simulink model "EV3_pos_control"  (Simulink 9.2)
settings: Solver=FixedStepDiscrete  StartTime=0.0  StopTime=Inf  RelTol=1e-3  EnableMultiTasking=on
InitFcn:
  | nxt_rst
values from neighbouring files (symbols this model uses):
  R = double(vpa(coeffs(collect(expand(eval(Ax*R0))),z_),Acc))    [nxt_rst.m]
  S = double(vpa(coeffs(collect(expand(eval((1-z_)^p*Bx*S2))),z_),Acc))    [nxt_rst.m]
  T = double(vpa(coeffs(collect(expand(eval(Ax*T0))),z_),Acc))    [nxt_rst.m]
  Te = 0.01    [init_ident.m]    (also in nxt_rst.m)
undefined symbols (not defined in the file or in its folder): adjustCoefficients
libraries: rpi_blkst x1
settings Model: Creator=jacques  LastModifiedBy=jacques  SimulationMode=external
settings OptimizationCC: ExpressionDepthLimit=2147483647  LifeSpan=1
settings DebuggingCC: SolverPrmCheckMsg=warning
settings HardwareCC: ProdLargestAtomicInteger=Long  ProdLargestAtomicFloat=Double  ProdIntDivRoundTo=Zero  ProdEndianess=LittleEndian  ProdHWDeviceType=ARM Compatible->ARM Cortex
settings SFSimCC: MATLABDynamicMemAlloc=off
settings RTWCC: SystemTargetFile=ert_rpi.tlc  TemplateMakefile=ert_rpi.tmf  PostCodeGenCommand=postGenFunc(buildInfo)  Description=RTW Embedded Coder RPI target
settings CodeAppCC: IgnoreCustomStorageClasses=off  CustomSymbolStrType=$N$R$M  InternalIdentifier=Classic
settings STFCustomTargetCC: ModelReferenceCompliant=off  CombineOutputUpdateFcns=on  ERTCustomFileBanners=on  SupportNonInlinedSFcns=off  RemoveResetFunc=on  MATLABClassNameForMDSCustomization=Simulink.SoftwareTarget.ERTCustomization  GRTInterface=off  SystemTargetFile=ert_rpi.tlc
settings ERTTargetCC: MultiwordLength=2048  ModelReferenceCompliant=off  ParMdlRefBuildCompliant=off  CompOptLevelCompliant=off  ConcurrentExecutionCompliant=off  SupportContinuousTime=on  ModelStepFunctionPrototypeControlCompliant=off  CPPClassGenCompliant=off  UseToolchainInfoCompliant=off  ExtMode=on  ExtModeMexArgs='192.168.2.1'  ERTCustomFileTemplate=ert_rpi_file_process.tlc  ConvertIfToSwitch=off  SuppressUnreachableDefaultCases=off

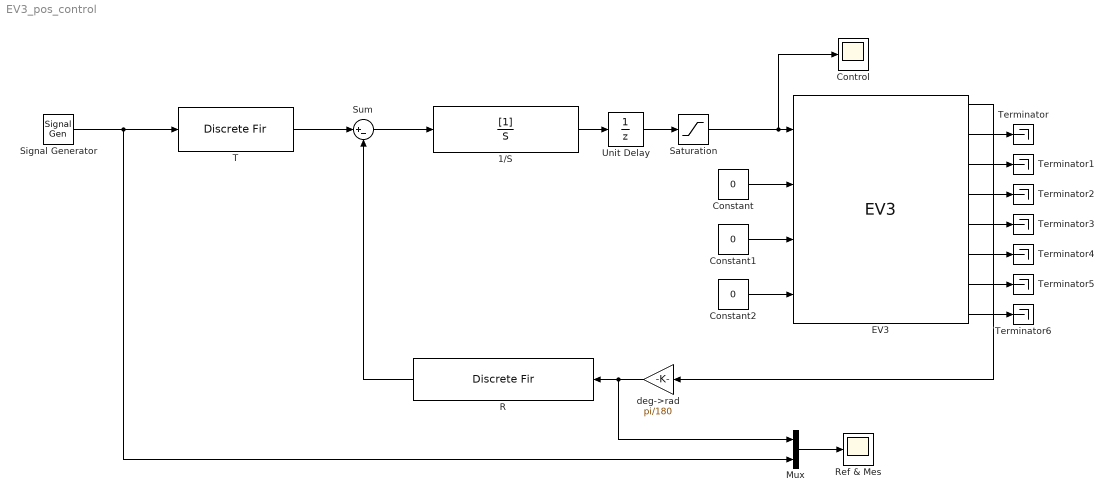
== system EV3_pos_control ==
  1/S : DiscreteFilter  Denominator=S  SampleTime=Te
  Constant : Constant  Value=0  SampleTime=0.01
  Constant1 : Constant  Value=0  SampleTime=0.01
  Constant2 : Constant  Value=0  SampleTime=0.01
  Control : Scope
  EV3 : rpi_blkst/EV3  rpi_mask_Ts=Te
      settings: SourceProductName=RPI Blockset
  Mux : Mux  Inputs=2
  R : DiscreteFir  Coefficients=adjustCoefficients(R)  SampleTime=Te  AccumDataTypeStr=Inherit: Same as product output
  Ref & Mes : Scope
  Saturation : Saturate  UpperLimit=100  LowerLimit=-100  SampleTime=Te
  Signal Generator : SignalGenerator  Frequency=0.5
  Sum : Sum  Inputs=|+-  SampleTime=Te
  T : DiscreteFir  Coefficients=adjustCoefficients(T)  SampleTime=Te  AccumDataTypeStr=Inherit: Same as product output
  Terminator{,1..6} (7 alike) : Terminator
  Unit Delay : UnitDelay  SampleTime=Te
  deg->rad : Gain  Gain=pi/180  SampleTime=Te
  wires:
  T/1 -> Sum/1
  R/1 -> Sum/2
  deg->rad/1 -> R/1, Mux/1
  1/S/1 -> Unit Delay/1
  Saturation/1 -> Control/1, EV3/1
  EV3/1 -> deg->rad/1
  Signal Generator/1 -> Mux/2, T/1
  EV3/2 -> Terminator/1
  EV3/3 -> Terminator1/1
  EV3/4 -> Terminator2/1
  EV3/5 -> Terminator3/1
  EV3/6 -> Terminator4/1
  EV3/7 -> Terminator5/1
  EV3/8 -> Terminator6/1
  Constant/1 -> EV3/2
  Constant1/1 -> EV3/3
  Constant2/1 -> EV3/4
  Mux/1 -> Ref & Mes/1
  Unit Delay/1 -> Saturation/1
  Sum/1 -> 1/S/1
